simulink library "governor_lib"  (R2022b)
settings: Solver=VariableStepAuto  StartTime=0.0  StopTime=10.0  RelTol=1e-3
settings Model: Creator=dr_pa  LastModifiedBy=dr_pa

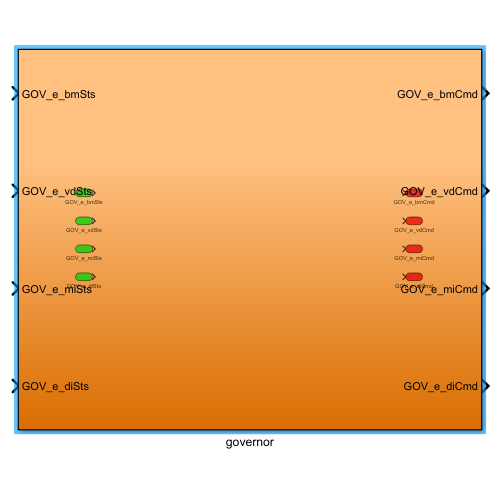
[thumbnail: Simulink's stored preview of the top-level diagram]
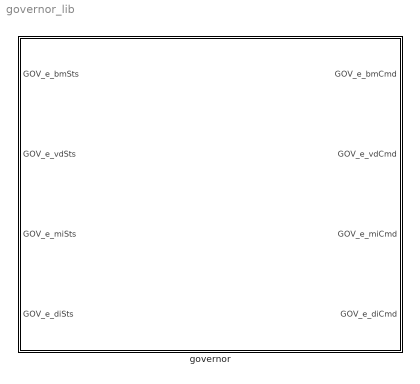
== system governor_lib ==
  governor : Subsystem

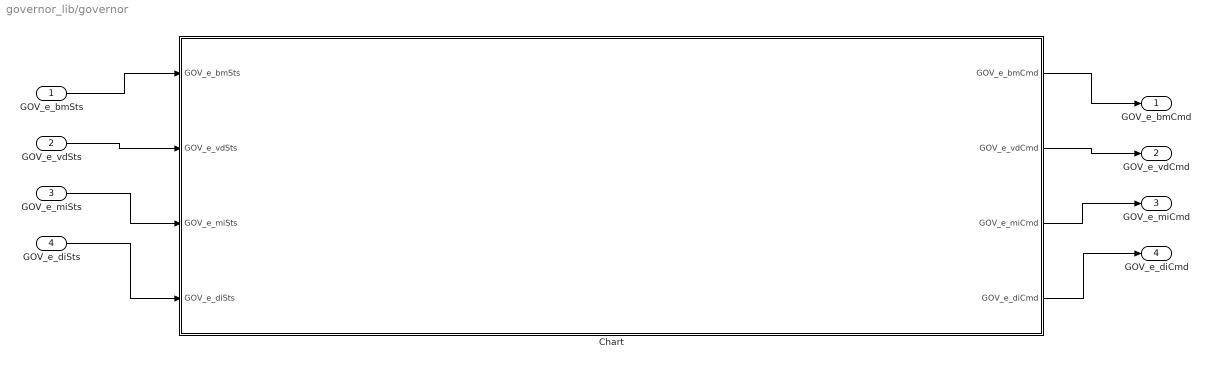
== system governor_lib/governor ==
  GOV_e_bmSts : Inport
  GOV_e_vdSts : Inport  Port=2
  GOV_e_miSts : Inport  Port=3
  GOV_e_diSts : Inport  Port=4
  Chart : Stateflow chart  TreatAsAtomicUnit=on
  GOV_e_bmCmd : Outport
  GOV_e_vdCmd : Outport  Port=2
  GOV_e_miCmd : Outport  Port=3
  GOV_e_diCmd : Outport  Port=4
  wires:
  GOV_e_bmSts/1 -> Chart/1(GOV_e_bmSts)
  GOV_e_vdSts/1 -> Chart/2(GOV_e_vdSts)
  GOV_e_miSts/1 -> Chart/3(GOV_e_miSts)
  GOV_e_diSts/1 -> Chart/4(GOV_e_diSts)
  Chart/1(GOV_e_bmCmd) -> GOV_e_bmCmd/1
  Chart/2(GOV_e_vdCmd) -> GOV_e_vdCmd/1
  Chart/3(GOV_e_miCmd) -> GOV_e_miCmd/1
  Chart/4(GOV_e_diCmd) -> GOV_e_diCmd/1

== stateflow chart governor_lib/governor/Chart ==
  state Vehicle_startup [group]
    state Initialize_outputs
      en:
      GOV_e_bmCmd = BM_IDLE
      GOV_e_vdCmd = VD_IDLE
      GOV_e_miCmd = MI_IDLE
      GOV_e_diCmd = DI_IDLE
    state init_mi_waitingForCAN
      % wait for motor interface to report
      % CAN success
      en:
    state init_mi_initialize
      % initialize motor controller?
      en:
    state init_bm_waitingForCAN
      % initialize motor controller?
      en:
    state init_waitingForPG6
      % initialize motor controller?
      en:
    state init_mi_CANinitError
      % wait for motor interface to report
      % CAN success
      en:
      % turn on LED? PA5?
    state init_bm_CANinitError
      % wait for motor interface to report
      % CAN success
      en:
      % turn on LED? PA5?
    Initialize_outputs -> init_mi_waitingForCAN
    init_mi_waitingForCAN -> init_mi_initialize [order 1] : [GOV_e_miSts == MI_CANactive]
    init_mi_initialize -> init_bm_waitingForCAN
    init_bm_waitingForCAN -> init_waitingForPG6 [order 1] : [GOV_e_biSts == BM_CANactive]
        | {% set status LED, PA5?}
    init_mi_waitingForCAN -> init_mi_CANinitError [order 2] : [GOV_e_miSts == MI_CANerr]
    init_bm_waitingForCAN -> init_bm_CANinitError [order 2]
  (default) -> Initialize_outputs
  data: GOV_e_bmSts input; GOV_e_vdSts input; GOV_e_miSts input; GOV_e_diSts input; GOV_e_bmCmd output; GOV_e_vdCmd output; GOV_e_miCmd output; GOV_e_diCmd output
